simulink model "Integrate1_Steering2Turn"  (R2021b)
settings: Solver=FixedStepAuto  StartTime=0.0  StopTime=inf  FixedStep=0.01  RelTol=1e-3
libraries: arduinolib x4
settings Model: ExtModeTrigDuration=2  Creator=user  LastModifiedBy=user
settings OptimizationCC: EnhancedBackFolding=on  PassReuseOutputArgsAs=Individual arguments  ZeroExternalMemoryAtStartup=off  ZeroInternalMemoryAtStartup=off  MaxStackSize=64  OptimizeBlockOrder=speed  DifferentSizesBufferReuse=on  OptimizationCustomize=off  EfficientTunableParamExpr=on
settings DebuggingCC: ParameterTunabilityLossMsg=error  UnconnectedInputMsg=none  UnconnectedOutputMsg=none  UnconnectedLineMsg=none
settings HardwareCC: ProdBitPerInt=16  ProdBitPerPointer=16  ProdBitPerSizeT=16  ProdBitPerPtrDiffT=16  ProdLargestAtomicFloat=None  ProdWordSize=8  ProdHWDeviceType=Atmel->AVR
settings ModelReferenceCC: EnableRefExpFcnMdlSchedulingChecks=off
settings SFSimCC: MATLABDynamicMemAlloc=off
settings RTWCC: Description=Embedded Coder  SystemTargetFile=ert.tlc  HardwareBoard=Arduino Uno  TemplateMakefile=ert_default_tmf  Toolchain=Arduino AVR  BuildConfiguration=Faster Runs  DLArmComputeVersion=20.02.1
settings CodeAppCC: ForceParamTrailComments=on  IgnoreCustomStorageClasses=off  OperatorAnnotations=on  SimulinkDataObjDesc=on  SFDataObjDesc=on  InsertBlockDesc=on
settings ERTTargetCC: SupportContinuousTime=on  SupportVariableSizeSignals=on  ExtModeTransport=3  ExtModeStaticAlloc=on  ExtModeStaticAllocSize=250  ExtModeMexFile=ext_xcp  ExtModeIntrfLevel=Level2 - Open

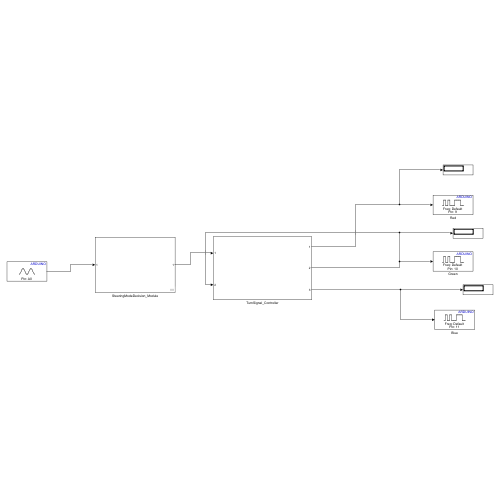
[thumbnail: Simulink's stored preview of the top-level diagram]
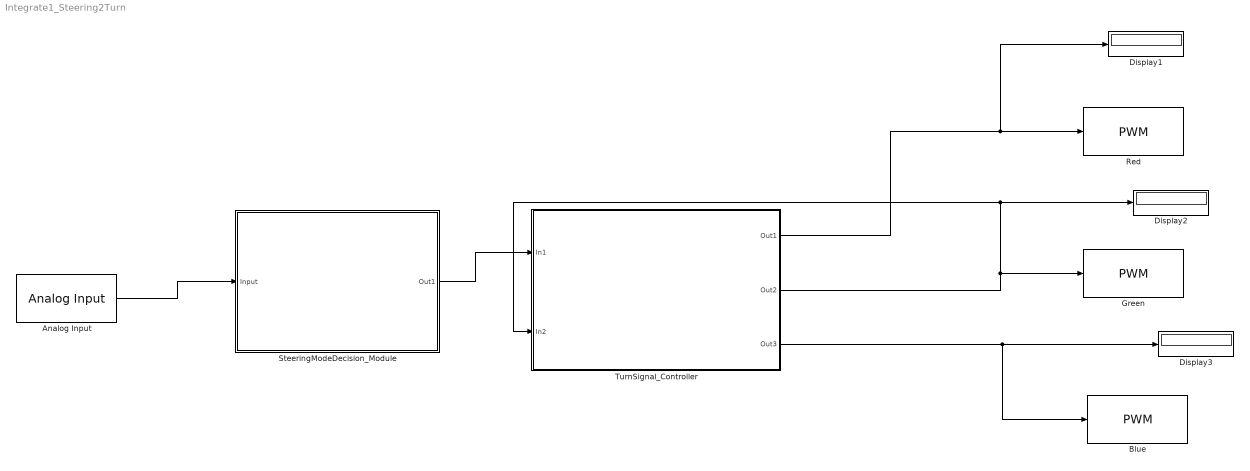
== system Integrate1_Steering2Turn ==
  Analog Input : arduinolib/Analog Input  pinNumber=0  ReadResultsOnly=off  ConversionTriggerSource=Software  ExternalTriggerType=uint32( 0 )  OutputDataType=uint16  EnableConversionCompleteNotify=off  EnableOuputStatus=off  SampleTime=-1  blockPlatform=arduino
  Blue : arduinolib/PWM  pinNumber=11  frequencyType=Default  desiredFrequency=490.2  achievableFrequency=490.2
  Display1 : Display
  Display2 : Display
  Display3 : Display
  Green : arduinolib/PWM  pinNumber=10  frequencyType=Default  desiredFrequency=490.2  achievableFrequency=490.2
  Red : arduinolib/PWM  pinNumber=9  frequencyType=Default  desiredFrequency=490.2  achievableFrequency=490.2
  SteeringModeDecision_Module : Subsystem
  TurnSignal_Controller : Subsystem
  wires:
  TurnSignal_Controller/1(Out1) -> Display1/1, Red/1
  TurnSignal_Controller/2(Out2) -> TurnSignal_Controller/2(In2), Display2/1, Green/1
  TurnSignal_Controller/3(Out3) -> Blue/1, Display3/1
  Analog Input/1 -> SteeringModeDecision_Module/1(Input)
  SteeringModeDecision_Module/1(Out1) -> TurnSignal_Controller/1(In1)

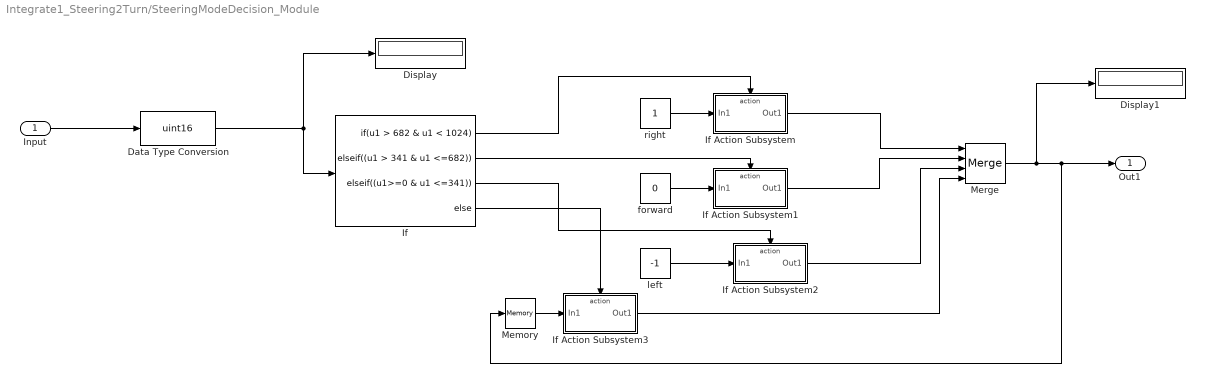
== system Integrate1_Steering2Turn/SteeringModeDecision_Module ==
  Input : Inport
  Data Type Conversion : DataTypeConversion  OutDataTypeStr=uint16
  Display : Display
  Display1 : Display
  If : If  IfExpression=u1 > 682 & u1 < 1024  ElseIfExpressions=(u1 > 341 & u1 <=682),(u1>=0 & u1 <=341)
  If Action Subsystem : Subsystem  TreatAsAtomicUnit=on
  If Action Subsystem1 : Subsystem  TreatAsAtomicUnit=on
  If Action Subsystem2 : Subsystem  TreatAsAtomicUnit=on
  If Action Subsystem3 : Subsystem  TreatAsAtomicUnit=on
  Memory : Memory
  Merge : Merge  Inputs=4
  forward : Constant  Value=0  OutDataTypeStr=double
  left : Constant  Value=-1  OutDataTypeStr=double
  right : Constant  OutDataTypeStr=double
  Out1 : Outport
  wires:
  If Action Subsystem2/1(Out1) -> Merge/3
  If/1 -> If Action Subsystem/Action
  left/1 -> If Action Subsystem2/1(In1)
  forward/1 -> If Action Subsystem1/1(In1)
  If/2 -> If Action Subsystem1/Action
  If Action Subsystem/1(Out1) -> Merge/1
  If Action Subsystem1/1(Out1) -> Merge/2
  right/1 -> If Action Subsystem/1(In1)
  Merge/1 -> Display1/1, Memory/1, Out1/1
  Input/1 -> Data Type Conversion/1
  Data Type Conversion/1 -> If/1, Display/1
  If/3 -> If Action Subsystem2/Action
  If/4 -> If Action Subsystem3/Action
  Memory/1 -> If Action Subsystem3/1(In1)
  If Action Subsystem3/1(Out1) -> Merge/4

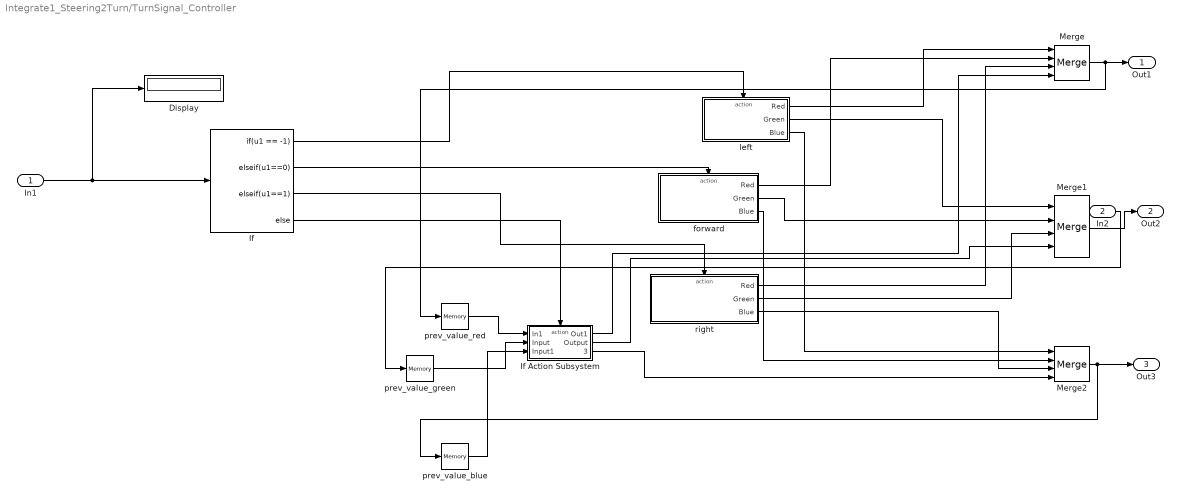
== system Integrate1_Steering2Turn/TurnSignal_Controller ==
  In1 : Inport
  In2 : Inport  Port=2
  Display : Display
  If : If  IfExpression=u1 == -1  ElseIfExpressions=u1==0, u1==1
  If Action Subsystem : Subsystem  TreatAsAtomicUnit=on
  Merge : Merge  Inputs=4
  Merge1 : Merge  Inputs=4
  Merge2 : Merge  Inputs=4
  forward : Subsystem  TreatAsAtomicUnit=on
  left : Subsystem  TreatAsAtomicUnit=on
  prev_value_blue : Memory  InheritSampleTime=on
  prev_value_green : Memory  InheritSampleTime=on
  prev_value_red : Memory  InheritSampleTime=on
  right : Subsystem  TreatAsAtomicUnit=on
  Out1 : Outport
  Out2 : Outport  Port=2
  Out3 : Outport  Port=3
  wires:
  forward/3(Blue) -> Merge2/2
  In1/1 -> If/1, Display/1
  right/2(Green) -> Merge1/3
  If/2 -> forward/Action
  prev_value_blue/1 -> If Action Subsystem/3(Input1)
  right/1(Red) -> Merge/3
  right/3(Blue) -> Merge2/3
  If/4 -> If Action Subsystem/Action
  forward/1(Red) -> Merge/2
  left/2(Green) -> Merge1/1
  forward/2(Green) -> Merge1/2
  If Action Subsystem/1(Out1) -> Merge/4
  Merge/1 -> Out1/1, prev_value_red/1
  Merge2/1 -> Out3/1, prev_value_blue/1
  left/1(Red) -> Merge/1
  If/3 -> right/Action
  In2/1 -> prev_value_green/1
  prev_value_green/1 -> If Action Subsystem/2(Input)
  prev_value_red/1 -> If Action Subsystem/1(In1)
  left/3(Blue) -> Merge2/1
  If Action Subsystem/3(Output1) -> Merge2/4
  If/1 -> left/Action
  If Action Subsystem/2(Output) -> Merge1/4
  Merge1/1 -> Out2/1

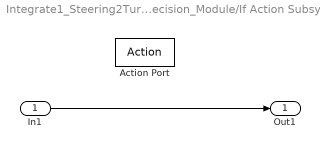
== system Integrate1_Steering2Turn/SteeringModeDecision_Module/If Action Subsystem ==
  In1 : Inport
  Action Port : ActionPort
  Out1 : Outport
  wires:
  In1/1 -> Out1/1

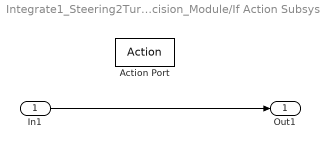
== system Integrate1_Steering2Turn/SteeringModeDecision_Module/If Action Subsystem1 ==
  In1 : Inport
  Action Port : ActionPort
  Out1 : Outport
  wires:
  In1/1 -> Out1/1

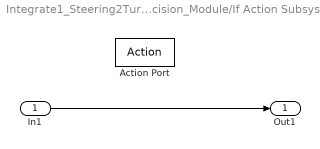
== system Integrate1_Steering2Turn/SteeringModeDecision_Module/If Action Subsystem2 ==
  In1 : Inport
  Action Port : ActionPort
  Out1 : Outport
  wires:
  In1/1 -> Out1/1

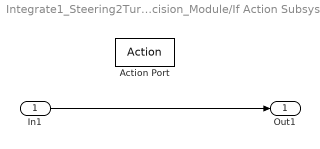
== system Integrate1_Steering2Turn/SteeringModeDecision_Module/If Action Subsystem3 ==
  In1 : Inport
  Action Port : ActionPort
  Out1 : Outport
  wires:
  In1/1 -> Out1/1

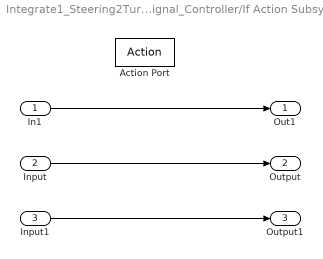
== system Integrate1_Steering2Turn/TurnSignal_Controller/If Action Subsystem ==
  In1 : Inport
  Input : Inport  Port=2
  Input1 : Inport  Port=3
  Action Port : ActionPort  ActionPortLabel=else
  Out1 : Outport
  Output : Outport  Port=2
  Output1 : Outport  Port=3
  wires:
  In1/1 -> Out1/1
  Input/1 -> Output/1
  Input1/1 -> Output1/1

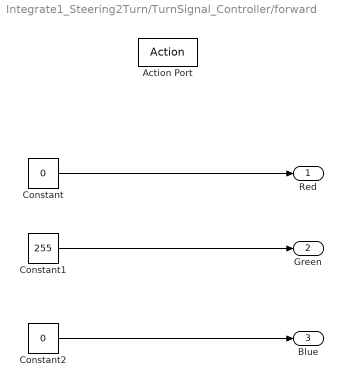
== system Integrate1_Steering2Turn/TurnSignal_Controller/forward ==
  Action Port : ActionPort  ActionPortLabel=elseif(u1==0)
  Constant : Constant  Value=0
  Constant1 : Constant  Value=255
  Constant2 : Constant  Value=0
  Red : Outport
  Green : Outport  Port=2
  Blue : Outport  Port=3
  wires:
  Constant2/1 -> Blue/1
  Constant1/1 -> Green/1
  Constant/1 -> Red/1

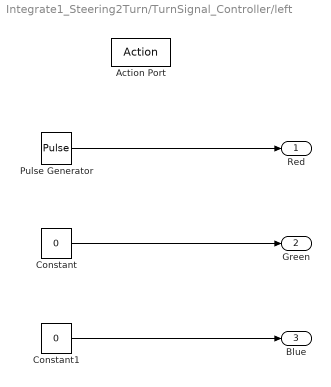
== system Integrate1_Steering2Turn/TurnSignal_Controller/left ==
  Action Port : ActionPort  ActionPortLabel=if(u1 == -1)
  Constant : Constant  Value=0
  Constant1 : Constant  Value=0
  Pulse Generator : DiscretePulseGenerator  Amplitude=255  Period=100  PulseWidth=50  SampleTime=-1
  Red : Outport
  Green : Outport  Port=2
  Blue : Outport  Port=3
  wires:
  Pulse Generator/1 -> Red/1
  Constant/1 -> Green/1
  Constant1/1 -> Blue/1

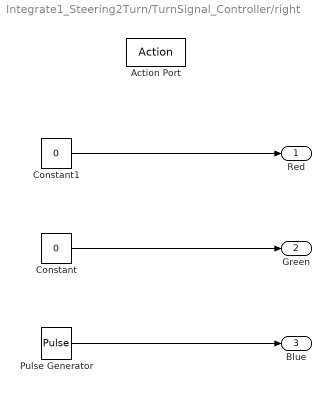
== system Integrate1_Steering2Turn/TurnSignal_Controller/right ==
  Action Port : ActionPort  ActionPortLabel=elseif( u1==1)
  Constant : Constant  Value=0
  Constant1 : Constant  Value=0
  Pulse Generator : DiscretePulseGenerator  Amplitude=255  Period=100  PulseWidth=50  SampleTime=-1
  Red : Outport
  Green : Outport  Port=2
  Blue : Outport  Port=3
  wires:
  Constant1/1 -> Red/1
  Pulse Generator/1 -> Blue/1
  Constant/1 -> Green/1
